simulink model "addviewer_floatingscope"  (R2022a)
settings: Solver=VariableStepAuto  StartTime=0.0  StopTime=10  RelTol=1e-3
settings Model: Creator=Home computer  LastModifiedBy=Home computer

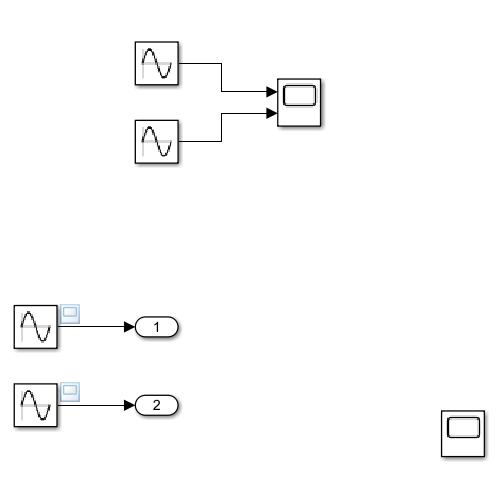
[thumbnail: Simulink's stored preview of the top-level diagram]
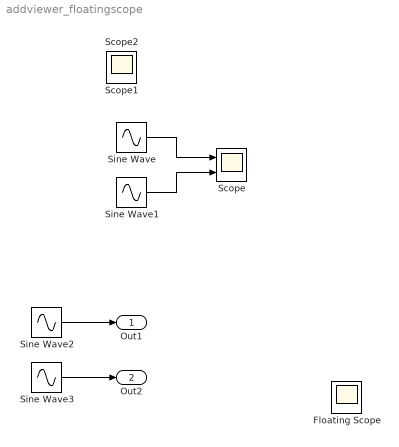
== system addviewer_floatingscope ==
  Floating Scope : Scope
      settings: Floating=on
  Scope : Scope  NumInputPorts=2
  Sine Wave : Sin  Amplitude=5  SampleTime=0
  Sine Wave1 : Sin  Amplitude=2  SampleTime=0
  Sine Wave2 : Sin  Amplitude=3  SampleTime=0
  Sine Wave3 : Sin  Amplitude=4  SampleTime=0
  Out1 : Outport
  Out2 : Outport  Port=2
  Scope1 : Scope
  Scope2 : Scope
  wires:
  Sine Wave/1 -> Scope/1
  Sine Wave1/1 -> Scope/2
  Sine Wave2/1 -> Out1/1
  Sine Wave3/1 -> Out2/1
